simulink model "EPS_sim_test_v4_R19a"  (R2019a)
settings: Solver=FixedStepAuto  StartTime=0.0  StopTime=tsimulation  FixedStep=delta_t  MaxStep=10  RelTol=1e-3
values from neighbouring files (symbols this model uses):
  C = Cbat*Nbp*3600    (= 37440)    [demoEPS.m]    (also in demoEPS_R2019a.m; demoEPS_v1.m; demoEPS_v1a.m; demoEPS_v1test.m)
  DOD_0 = 0    [demoEPS.m]    (also in demoEPS_R2019a.m; demoEPS_v1.m; demoEPS_v1a.m; demoEPS_v1test.m)
  eff_iBat = 0.95    [demoEPS_v3.m]    (also in demoEPS_v4.m; demoEPS_v5.m)
  I_BC_max = -input (4)    [battchargedischarge.m]    (also in demoEPS.m = 3; demoEPS_R2019a.m = 3; demoEPS_v1.m = 3; demoEPS_v1a.m = 3)
  I_BD_max = input (3)    [battchargedischarge.m]    (also in demoEPS.m = 5; demoEPS_R2019a.m = 5; demoEPS_v1.m = 5; demoEPS_v1a.m = 5)
  Nbs = math.ceil(Vbusmin/Vbatmin)    [calc_mass_EPS.m]    (also in demoEPS.m = 4; demoEPS_R2019a.m = 4; demoEPS_v1.m = 4; demoEPS_v1a.m = 4)
  P_eps = 0.6    [demoEPS.m]    (also in demoEPS_R2019a.m; demoEPS_v1.m; demoEPS_v1a.m; demoEPS_v1test.m)
  Psa = 48    [demoEPS.m]    (also in demoEPS_R2019a.m; demoEPS_v1.m; demoEPS_v1a.m; demoEPS_v1test.m)
  Torb = 2*pi*sqrt(a^3/(3.986004418E5))    [demoEPS_v4.m]    (also in demoEPS_v5.m)
libraries: simulink x3
settings Model: Creator=Ricardo  LastModifiedBy=arami

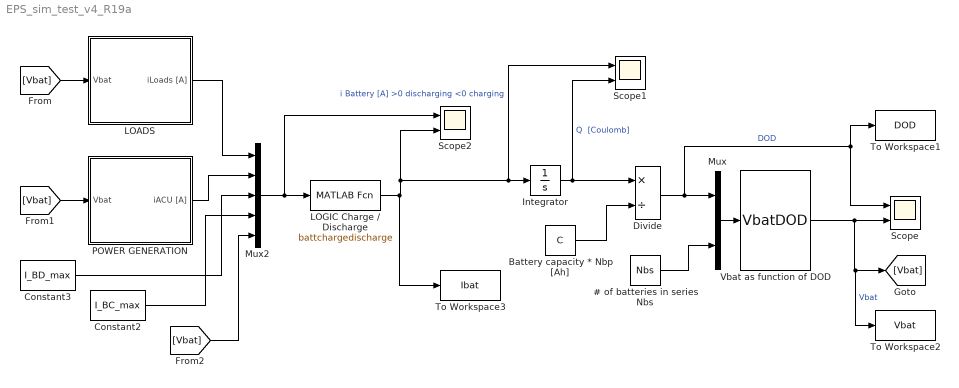
== system EPS_sim_test_v4_R19a ==
  # of batteries in series Nbs : Constant  Value=Nbs
  Battery capacity * Nbp [Ah] : Constant  Value=C
  Constant2 : Constant  Value=I_BC_max
  Constant3 : Constant  Value=I_BD_max
  Divide : Product  Inputs=*/
  Integrator : Integrator  InitialCondition=DOD_0
  LOADS : Subsystem
  LOGIC Charge / Discharge : MATLABFcn  MATLABFcn=battchargedischarge
  Mux : Mux  Inputs=2
  Mux2 : Mux  Inputs=5
  POWER GENERATION : Subsystem
  Scope : Scope  NumInputPorts=2
  Scope1 : Scope  NumInputPorts=2
  Scope2 : Scope  NumInputPorts=2
  To Workspace1 : ToWorkspace  VariableName=DOD  SaveFormat=Timeseries  SampleTime=-1
  To Workspace2 : ToWorkspace  VariableName=Vbat  SaveFormat=Timeseries  SampleTime=-1
  To Workspace3 : ToWorkspace  VariableName=Ibat  SaveFormat=Timeseries  SampleTime=-1
  Vbat as function of DOD : MATLABFcn  MATLABFcn=VbatDOD
  wires:
  Mux/1 -> Vbat as function of DOD/1
  # of batteries in series Nbs/1 -> Mux/2
  Vbat as function of DOD/1 -> To Workspace2/1, [Vbat], Scope/2  "Vbat"
  Divide/1 -> To Workspace1/1, Scope/1, Mux/1  "DOD"
  Integrator/1 -> Scope1/2, Divide/1  "Q  [Coulomb]"
  Battery capacity * Nbp [Ah]/1 -> Divide/2
  [Vbat] -> LOADS/1(Vbat)
  POWER GENERATION/1(iACU [A]) -> Mux2/2
  [Vbat] -> POWER GENERATION/1(Vbat)
  LOADS/1(iLoads [A]) -> Mux2/1
  Mux2/1 -> LOGIC Charge / Discharge/1, Scope2/1
  Constant3/1 -> Mux2/3
  Constant2/1 -> Mux2/4
  LOGIC Charge / Discharge/1 -> To Workspace3/1, Scope1/1, Integrator/1, Scope2/2  "i Battery [A] >0 discharging <0 charging"
  [Vbat] -> Mux2/5

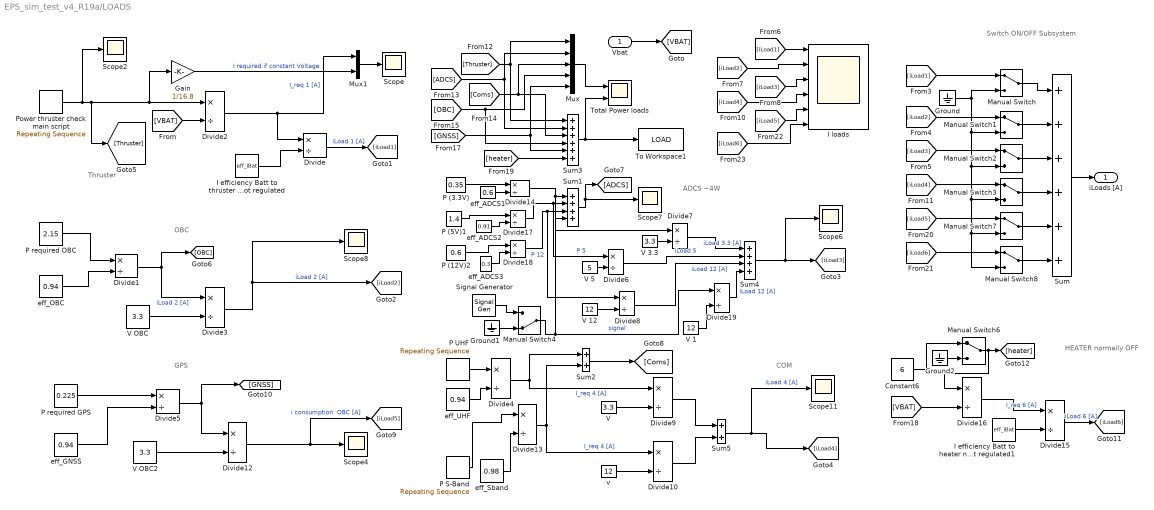
== system EPS_sim_test_v4_R19a/LOADS ==
  note: Switch
      | ON/OFF
      | Subsystem
  note: Thruster
  note: OBC
  note: ADCS ~4W
  note: COM
  note: GPS
  note: HEATER
      | normally
      | OFF
  Vbat : Inport
  Constant6 : Constant  Value=6
  Divide{,1..10,12..19} (19 alike) : Product  Inputs=*/
  Gain : Gain  Gain=1/16.8
  Ground : Ground
  Ground1 : Ground
  Ground2 : Ground
  I efficiency Batt to heater not regulated1 : Constant  Value=eff_iBat
  I efficiency Batt to thruster not regulated : Constant  Value=eff_iBat
  I loads : Scope  NumInputPorts=6
  Manual Switch{,1..3,6..8} (7 alike) : ManualSwitch
  Manual Switch4 : ManualSwitch  CurrentSetting=0
  Mux : Mux  Inputs=5
  Mux1 : Mux  Inputs=2
  P (12V)2 : Constant  Value=0.6
  P (3.3V) : Constant  Value=0.35
  P (5V)1 : Constant  Value=1.4
  P S-Band : simulink/Sources/Repeating Sequence  rep_seq_t=0  rep_seq_y=2.7
  "P UHF " : simulink/Sources/Repeating Sequence  rep_seq_t=0  rep_seq_y=2.7
  P required GPS : Constant  Value=0.225
  P required OBC : Constant  Value=2.15
  Power thruster check main script : simulink/Sources/Repeating Sequence  rep_seq_t=t_thr  rep_seq_y=p_thr
  Scope{,2,4,6..8,11} (7 alike) : Scope
  Signal Generator : SignalGenerator  WaveForm=random  Amplitude=0.6  Frequency=0.01
  Sum : Sum  Inputs=++++++
  Sum1 : Sum  Inputs=++++
  Sum2 : Sum
  Sum3 : Sum  Inputs=++++++
  Sum4 : Sum  Inputs=++++
  Sum5 : Sum
  To Workspace1 : ToWorkspace  VariableName=LOAD  SaveFormat=Timeseries  SampleTime=-1
  Total Power loads : Scope  NumInputPorts=2
  "V " : Constant  Value=3.3
  V 1 : Constant  Value=12
  V 12 : Constant  Value=12
  V 3.3 : Constant  Value=3.3
  V 5 : Constant  Value=5
  V OBC : Constant  Value=3.3
  V OBC2 : Constant  Value=3.3
  "eff_ADCS1 " : Constant  Value=0.6
  eff_ADCS2 : Constant  Value=0.91
  "eff_ADCS3 " : Constant  Value=0.3
  eff_GNSS : Constant  Value=0.94
  eff_OBC : Constant  Value=0.94
  eff_Sband : Constant  Value=0.98
  eff_UHF : Constant  Value=0.94
  v : Constant  Value=12
  iLoads [A] : Outport  VectorParamsAs1DForOutWhenUnconnected=on
  wires:
  Gain/1 -> Mux1/2  "I required if constant Voltage"
  Divide2/1 -> Divide/1, Mux1/1  "I_req 1 [A]"
  V OBC/1 -> Divide3/2
  Vbat/1 -> [VBAT]
  [VBAT] -> Divide2/2
  Sum/1 -> iLoads [A]/1
  Mux1/1 -> Scope/1
  eff_OBC/1 -> Divide1/2
  Power thruster check main script/1 -> Scope2/1, [Thruster], Gain/1, Divide2/1
  I efficiency Batt to thruster not regulated/1 -> Divide/2
  Divide/1 -> [iLoad1]  "iLoad 1 [A]"
  V 3.3/1 -> Divide7/2
  Manual Switch/1 -> Sum/1
  Manual Switch1/1 -> Sum/2
  Manual Switch2/1 -> Sum/3
  [iLoad2] -> I loads/2
  [iLoad1] -> I loads/1
  [iLoad3] -> I loads/3
  Sum1/1 -> Scope7/1, [ADCS]
  P (3.3V)/1 -> Divide14/1
  Signal Generator/1 -> Manual Switch4/1
  Sum5/1 -> Scope11/1, [iLoad4]  "iLoad 4 [A]"
  [iLoad4] -> I loads/4
  Manual Switch3/1 -> Sum/4
  "P UHF "/1 -> Divide4/1
  [iLoad4] -> Manual Switch3/1
  [iLoad3] -> Manual Switch2/1
  [iLoad2] -> Manual Switch1/1
  [iLoad1] -> Manual Switch/1
  Ground/1 -> Manual Switch/2, Manual Switch8/2, Manual Switch7/2, Manual Switch3/2, Manual Switch2/2, Manual Switch1/2
  Ground1/1 -> Manual Switch4/2
  Mux/1 -> Total Power loads/1
  [Thruster] -> Sum3/1, Mux/1
  [ADCS] -> Sum3/2, Mux/2
  [Coms] -> Sum3/3, Mux/3
  [OBC] -> Sum3/4, Mux/4
  [heater] -> Sum3/6
  Sum3/1 -> Total Power loads/2, To Workspace1/1
  Divide12/1 -> [iLoad5], Scope4/1  "i consumption  OBC [A]"
  V OBC2/1 -> Divide12/2
  eff_GNSS/1 -> Divide5/2
  [GNSS] -> Sum3/5, Mux/5
  I efficiency Batt to heater not regulated1/1 -> Divide15/2
  Divide15/1 -> [iLoad6]  "iLoad 6 [A]"
  Constant6/1 -> Manual Switch6/1
  Divide16/1 -> Divide15/1  "I_req 6 [A]"
  [VBAT] -> Divide16/2
  Manual Switch6/1 -> Divide16/1, [heater]
  Ground2/1 -> Manual Switch6/2
  Manual Switch7/1 -> Sum/5
  Manual Switch8/1 -> Sum/6
  [iLoad6] -> Manual Switch8/1
  [iLoad5] -> Manual Switch7/1
  [iLoad5] -> I loads/5
  [iLoad6] -> I loads/6
  P (5V)1/1 -> Divide17/1
  P (12V)2/1 -> Divide18/1
  "eff_ADCS1 "/1 -> Divide14/2
  "eff_ADCS3 "/1 -> Divide18/2
  eff_ADCS2/1 -> Divide17/2
  Divide14/1 -> Divide7/1, Sum1/1
  Divide17/1 -> Divide6/1, Sum1/2  "P 5"
  Divide18/1 -> Divide8/1, Sum1/3  "P 12"
  Manual Switch4/1 -> Divide19/1, Sum1/4  "signal"
  V 5/1 -> Divide6/2
  V 12/1 -> Divide8/2
  Divide7/1 -> Sum4/1  "iLoad 3.3 [A]"
  Divide6/1 -> Sum4/2  "iLoad 5"
  Divide8/1 -> Sum4/3  "iLoad 12 [A]"
  Sum4/1 -> [iLoad3], Scope6/1
  V 1/1 -> Divide19/2
  Divide19/1 -> Sum4/4  "iLoad 12 [A]"
  P required OBC/1 -> Divide1/1
  Divide1/1 -> [OBC], Divide3/1  "iLoad 2 [A]"
  Divide3/1 -> Scope8/1, [iLoad2]  "iLoad 2 [A]"
  P required GPS/1 -> Divide5/1
  Divide5/1 -> [GNSS], Divide12/1
  P S-Band/1 -> Divide13/1
  eff_Sband/1 -> Divide13/2
  Divide4/1 -> Divide9/1, Sum2/1  "I_req 4 [A]"
  Divide13/1 -> Sum2/2, Divide10/1  "I_req 4 [A]"
  Sum2/1 -> [Coms]
  eff_UHF/1 -> Divide4/2
  "V "/1 -> Divide9/2
  v/1 -> Divide10/2
  Divide10/1 -> Sum5/2
  Divide9/1 -> Sum5/1

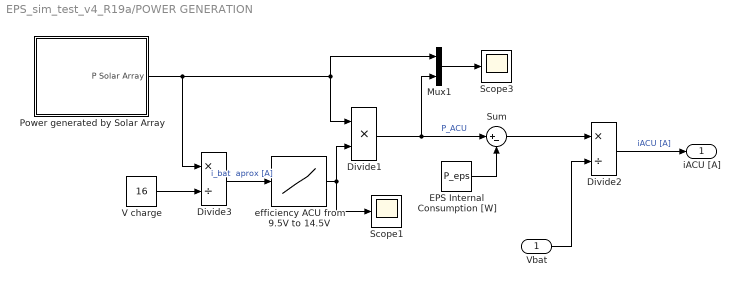
== system EPS_sim_test_v4_R19a/POWER GENERATION ==
  Vbat : Inport
  Divide1 : Product  Inputs=**
  Divide2 : Product  Inputs=*/
  Divide3 : Product  Inputs=*/
  EPS Internal Consumption [W] : Constant  Value=P_eps
  Mux1 : Mux  Inputs=2
  Power generated by Solar Array : Subsystem
  Scope1 : Scope
  Scope3 : Scope
  Sum : Sum  Inputs=|+-
  V charge : Constant  Value=16
  efficiency ACU from 9.5V to 14.5V : Lookup_n-D  NumberOfTableDimensions=1  BreakpointsForDimension1=[0,0.13,0.16,0.236,0.4187,0.654,0.684,0.745,0.801,0.9372,1.046,1.16,1.21,1.5,1.66,2,4]  Table=[0.905,0.928,0.9296,0.9296,0.9337,0.9296,0.9296,0.9296,0.9275,0.9275,0.9254,0.9254,0.9234,0.9193,0.9193,0.9134,0.9134]  InternalRulePriority=Speed  RndMeth=Simplest  InputSameDT=on
  iACU [A] : Outport  VectorParamsAs1DForOutWhenUnconnected=on
  wires:
  Divide2/1 -> iACU [A]/1  "iACU [A]"
  Mux1/1 -> Scope3/1
  Vbat/1 -> Divide2/2
  efficiency ACU from 9.5V to 14.5V/1 -> Scope1/1, Divide1/2
  Divide1/1 -> Sum/1, Mux1/2  "P_ACU"
  Sum/1 -> Divide2/1
  EPS Internal Consumption [W]/1 -> Sum/2
  Divide3/1 -> efficiency ACU from 9.5V to 14.5V/1  "i_bat  aprox [A]"
  V charge/1 -> Divide3/2
  Power generated by Solar Array/1(P Solar Array) -> Divide3/1, Divide1/1, Mux1/1

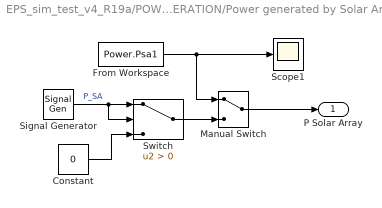
== system EPS_sim_test_v4_R19a/POWER GENERATION/Power generated by Solar Array ==
  Constant : Constant  Value=0
  From Workspace : FromWorkspace  VariableName=Power.Psa1  SampleTime=0
  Manual Switch : ManualSwitch
  Scope1 : Scope
  Signal Generator : SignalGenerator  Amplitude=-Psa  Frequency=1/Torb
  Switch : Switch  Criteria=u2 > Threshold
  P Solar Array : Outport  VectorParamsAs1DForOutWhenUnconnected=on
  wires:
  From Workspace/1 -> Manual Switch/1, Scope1/1
  Constant/1 -> Switch/3
  Signal Generator/1 -> Switch/2, Switch/1  "P_SA"
  Manual Switch/1 -> P Solar Array/1
  Switch/1 -> Manual Switch/2
